simulink model "SL_RC_shared_branch"  (R2026a)
settings: Solver=ode4  StopTime=4.0940000000000001e-06  FixedStep=1e-12  EnableMultiTasking=on
undefined symbols (not defined in the file): i, magnitude
settings Model: Creator=fxzhao  LastModifiedBy=35609
settings OptimizationCC: OptimizeBlockIOStorage=off  BufferReuse=off  GlobalBufferReuse=off  ExpressionFolding=off  LocalBlockOutputs=off
settings HardwareCC: ProdHWDeviceType=32-bit Generic

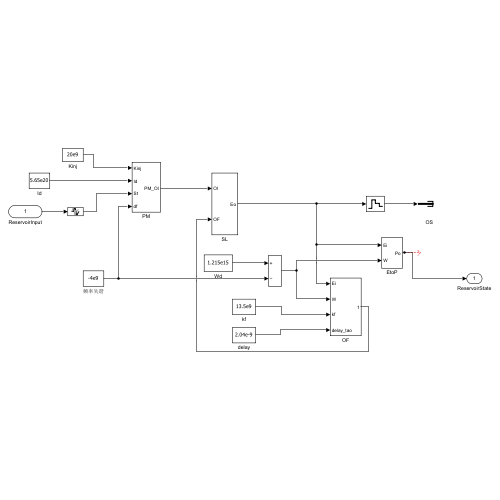
[thumbnail: Simulink's stored preview of the top-level diagram]
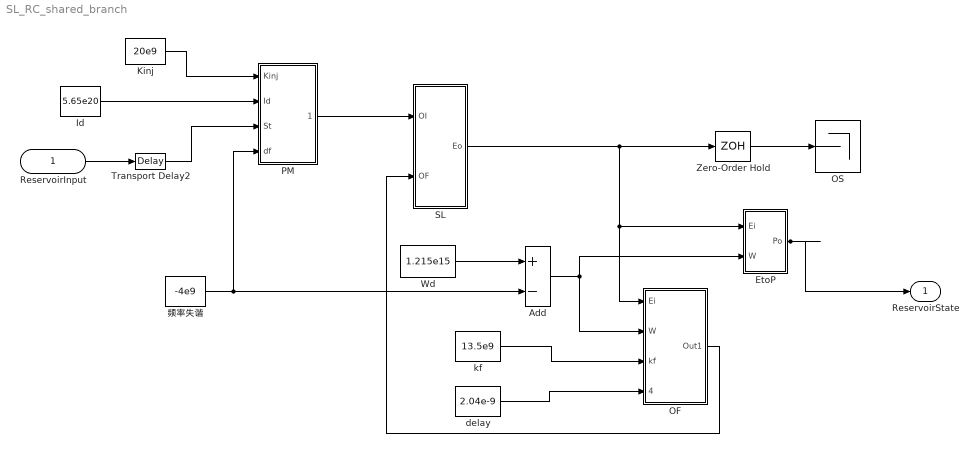
== system SL_RC_shared_branch ==
  ReservoirInput : Inport
  Add : Sum  Inputs=+-
  EtoP : Subsystem
  Id : Constant  Value=5.65e20
  "Kinj " : Constant  Value=20e9
  OF : Subsystem
  OS : Terminator
  PM : Subsystem
  "SL " : Subsystem
  Transport Delay2 : TransportDelay  DelayTime=4e-6  BufferSize=20000000
  Wd : Constant  Value=1.215e15
  Zero-Order Hold : ZeroOrderHold  SampleTime=1e-12
  delay : Constant  Value=2.04e-9  VectorParams1D=off
  kf : Constant  Value=13.5e9  VectorParams1D=off
  频率失谐 : Constant  Value=-4e9
  ReservoirState : Outport
  wires:
  kf/1 -> OF/3(kf)
  delay/1 -> OF/4(delay_tao)
  "SL "/1(Eo) -> Zero-Order Hold/1, OF/1(Ei), EtoP/1(Ei)
  频率失谐/1 -> Add/2, PM/4(df)
  Add/1 -> EtoP/2(W), OF/2(W)
  Wd/1 -> Add/1
  OF/1(Out1) -> "SL "/2(OF)
  EtoP/1(Po) -> ReservoirState/1
  "Kinj "/1 -> PM/1(Kinj)
  PM/1(PM_OI) -> "SL "/1(OI)
  Id/1 -> PM/2(Id)
  Transport Delay2/1 -> PM/3(St)
  Zero-Order Hold/1 -> OS/1
  ReservoirInput/1 -> Transport Delay2/1

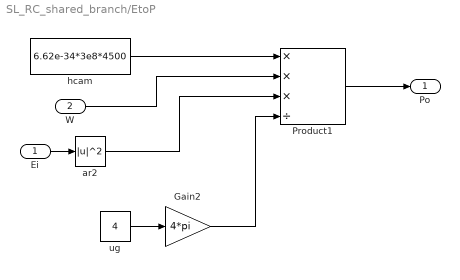
== system SL_RC_shared_branch/EtoP ==
  Ei : Inport
  W : Inport  Port=2
  Gain2 : Gain  Gain=4*pi
  Product1 : Product  Inputs=***/  RndMeth=Zero
  ar2 : Math  Operator=magnitude^2  SignedPower=on  OutputSignalType=real
  hcam : Constant  Value=6.62e-34*3e8*4500
  ug : Constant  Value=4
  Po : Outport
  wires:
  Ei/1 -> ar2/1
  ug/1 -> Gain2/1
  Product1/1 -> Po/1
  hcam/1 -> Product1/1
  W/1 -> Product1/2
  ar2/1 -> Product1/3
  Gain2/1 -> Product1/4

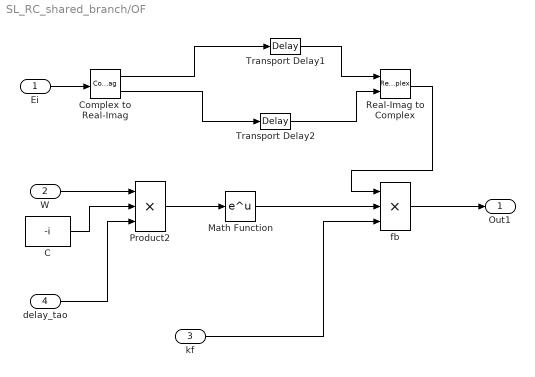
== system SL_RC_shared_branch/OF ==
  Ei : Inport
  W : Inport  Port=2
  kf : Inport  Port=3
  delay_tao : Inport  Port=4
  C : Constant  Value=-i  VectorParams1D=off
  Complex to Real-Imag : ComplexToRealImag
  Math Function : Math  SignedPower=on
  Product2 : Product  Inputs=3  RndMeth=Zero
  Real-Imag to Complex : RealImagToComplex
  Transport Delay1 : TransportDelay  DelayTime=2.04e-9  BufferSize=20000000
  Transport Delay2 : TransportDelay  DelayTime=2.04e-9  BufferSize=20000000
  fb : Product  Inputs=3  RndMeth=Zero
  Out1 : Outport
  wires:
  Math Function/1 -> fb/2
  Product2/1 -> Math Function/1
  fb/1 -> Out1/1
  W/1 -> Product2/1
  kf/1 -> fb/3
  Transport Delay1/1 -> Real-Imag to Complex/1
  Transport Delay2/1 -> Real-Imag to Complex/2
  Complex to Real-Imag/1 -> Transport Delay1/1
  Complex to Real-Imag/2 -> Transport Delay2/1
  Ei/1 -> Complex to Real-Imag/1
  Real-Imag to Complex/1 -> fb/1
  C/1 -> Product2/2
  delay_tao/1 -> Product2/3

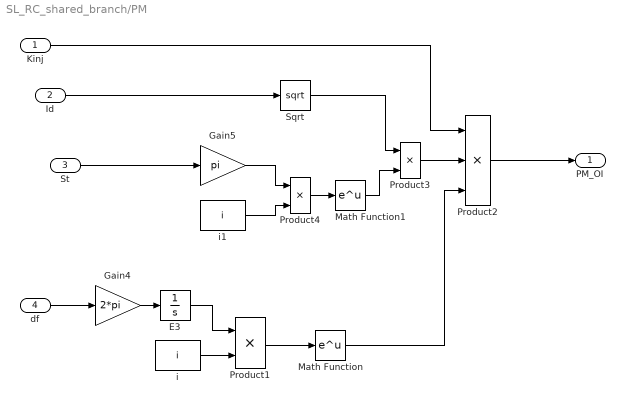
== system SL_RC_shared_branch/PM ==
  Kinj : Inport
  Id : Inport  Port=2
  St : Inport  Port=3
  df : Inport  Port=4
  E3 : Integrator  InitialCondition=1e-3
  Gain4 : Gain  Gain=2*pi
  Gain5 : Gain  Gain=pi
  Math Function : Math  SignedPower=on
  Math Function1 : Math  SignedPower=on
  Product1 : Product  RndMeth=Zero
  Product2 : Product  Inputs=3  RndMeth=Zero
  Product3 : Product  RndMeth=Zero
  Product4 : Product  RndMeth=Zero
  Sqrt : Sqrt
  i : Constant  Value=i  VectorParams1D=off
  i1 : Constant  Value=i  VectorParams1D=off
  PM_OI : Outport
  wires:
  Sqrt/1 -> Product3/1
  Math Function1/1 -> Product3/2
  i1/1 -> Product4/2
  Gain5/1 -> Product4/1
  Product4/1 -> Math Function1/1
  i/1 -> Product1/2
  E3/1 -> Product1/1
  Gain4/1 -> E3/1
  Product1/1 -> Math Function/1
  Kinj/1 -> Product2/1
  Product2/1 -> PM_OI/1
  Product3/1 -> Product2/2
  Math Function/1 -> Product2/3
  df/1 -> Gain4/1
  St/1 -> Gain5/1
  Id/1 -> Sqrt/1

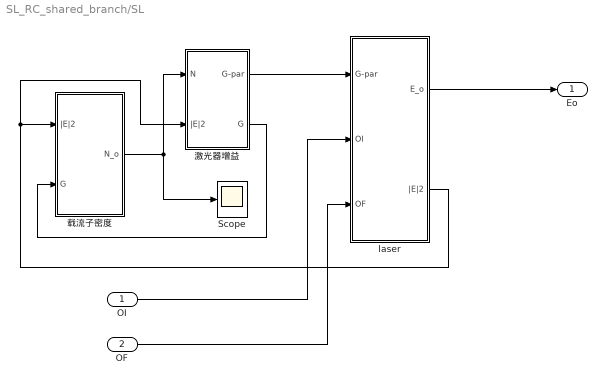
== system SL_RC_shared_branch/SL  ==
  OI : Inport
  OF : Inport  Port=2
  Scope : Scope
      settings: ActiveDisplayYMinimum=9.7171230843277208E+23  ActiveDisplayYMaximum=2.9717123084327718E+24  DataLoggingMaxPoints=10000  DataLoggingSaveFormat=Array
  laser : Subsystem
  激光器增益 : Subsystem
  载流子密度 : Subsystem
  Eo : Outport
  wires:
  激光器增益/2(G) -> 载流子密度/2(G)
  激光器增益/1(G-par) -> laser/1(G-par)
  laser/1(E_o) -> Eo/1
  laser/2(|E|2) -> 载流子密度/1(|E|2), 激光器增益/2(|E|2)
  载流子密度/1(N_o) -> Scope/1, 激光器增益/1(N)
  OI/1 -> laser/2(OI)
  OF/1 -> laser/3(OF)

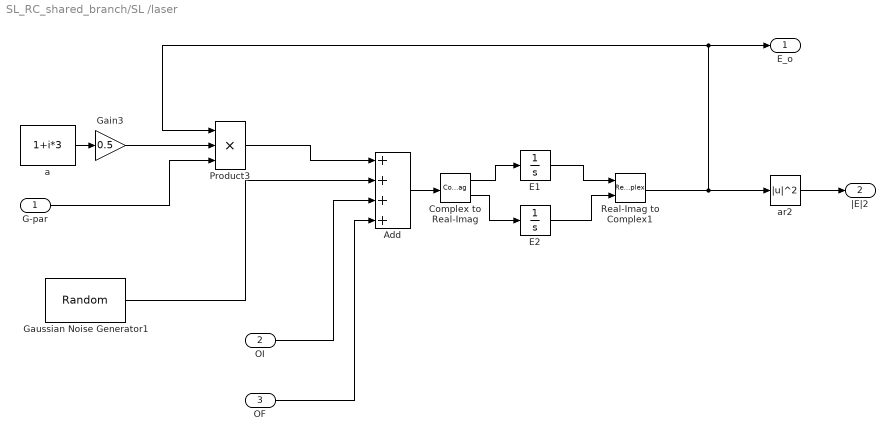
== system SL_RC_shared_branch/SL /laser ==
  G-par : Inport
  OI : Inport  Port=2
  OF : Inport  Port=3
  Add : Sum  Inputs=++++
  Complex to Real-Imag : ComplexToRealImag
  E1 : Integrator  InitialCondition=1e-3
  E2 : Integrator  InitialCondition=1e-3
  Gain3 : Gain  Gain=0.5
  Gaussian Noise Generator1 : RandomNumber  Variance=2.5e8  Seed=1  SampleTime=1e-12
  Product3 : Product  Inputs=3  RndMeth=Zero
  Real-Imag to Complex1 : RealImagToComplex
  a : Constant  Value=1+i*3
  ar2 : Math  Operator=magnitude^2  SignedPower=on  OutputSignalType=real
  E_o : Outport
  |E|2 : Outport  Port=2
  wires:
  G-par/1 -> Product3/3
  Gain3/1 -> Product3/2
  a/1 -> Gain3/1
  Product3/1 -> Add/1
  Real-Imag to Complex1/1 -> ar2/1, E_o/1, Product3/1
  ar2/1 -> |E|2/1
  Complex to Real-Imag/1 -> E1/1
  Complex to Real-Imag/2 -> E2/1
  E2/1 -> Real-Imag to Complex1/2
  Add/1 -> Complex to Real-Imag/1
  E1/1 -> Real-Imag to Complex1/1
  OI/1 -> Add/3
  OF/1 -> Add/4
  Gaussian Noise Generator1/1 -> Add/2

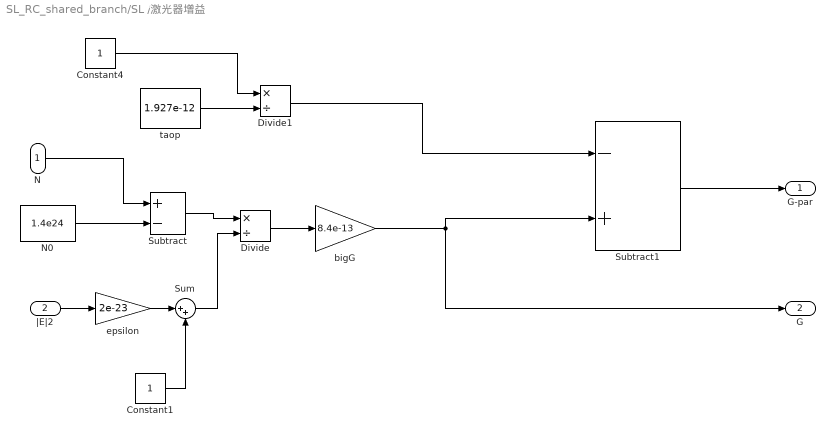
== system SL_RC_shared_branch/SL /激光器增益 ==
  N : Inport
  |E|2 : Inport  Port=2
  Constant1 : Constant
  Constant4 : Constant
  Divide : Product  Inputs=*/
  Divide1 : Product  Inputs=*/
  N0 : Constant  Value=1.4e24
  Subtract : Sum  Inputs=+-
  Subtract1 : Sum  Inputs=-+
  Sum : Sum  Inputs=|++
  bigG : Gain  Gain=8.4e-13
  epsilon : Gain  Gain=2e-23
  taop : Constant  Value=1.927e-12
  G-par : Outport
  G : Outport  Port=2
  wires:
  N0/1 -> Subtract/2
  epsilon/1 -> Sum/1
  Constant1/1 -> Sum/2
  Subtract/1 -> Divide/1
  Sum/1 -> Divide/2
  Divide/1 -> bigG/1
  bigG/1 -> G/1, Subtract1/2
  Subtract1/1 -> G-par/1
  taop/1 -> Divide1/2
  Constant4/1 -> Divide1/1
  N/1 -> Subtract/1
  Divide1/1 -> Subtract1/1
  |E|2/1 -> epsilon/1

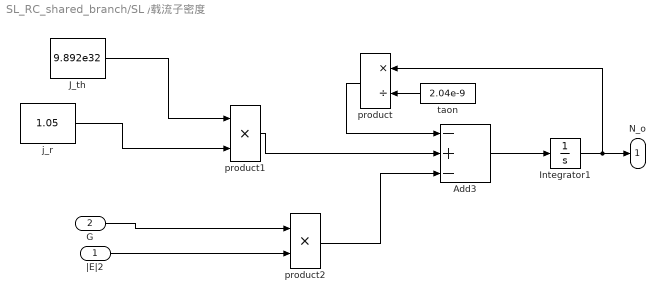
== system SL_RC_shared_branch/SL /载流子密度 ==
  |E|2 : Inport
  G : Inport  Port=2
  Add3 : Sum  Inputs=-+-
  Integrator1 : Integrator  InitialCondition=0.001  AbsoluteTolerance=1e-3
  J_th : Constant  Value=9.892e32
  j_r : Constant  Value=1.05
  product : Product  Inputs=*/  RndMeth=Zero
  product1 : Product  RndMeth=Zero
  product2 : Product  RndMeth=Zero
  taon : Constant  Value=2.04e-9
  N_o : Outport
  wires:
  G/1 -> product2/1
  |E|2/1 -> product2/2
  product2/1 -> Add3/3
  Add3/1 -> Integrator1/1
  Integrator1/1 -> product/1, N_o/1
  taon/1 -> product/2
  product1/1 -> Add3/2
  product/1 -> Add3/1
  J_th/1 -> product1/1
  j_r/1 -> product1/2
